simulink model "distmodelR2019a"  (R2019a)
settings: Solver=FixedStepAuto  StartTime=0.0  StopTime=t_sim  FixedStep=TimeStep  RelTol=1e-3
values from neighbouring files (symbols this model uses):
  alt = 300    [main_disturbances_Z.m]
  AX = 0.022    [calctorque.m]    (also in main_disturbances_Z.m)
  AY = 0.034    [calctorque.m]    (also in main_disturbances_Z.m)
  AZ = 0.0748    [calctorque.m]    (also in main_disturbances_Z.m = 0.2108)
  AZES = 0.1156    [calctorque.m]    (also in main_disturbances_Z.m)
  Cdrag = 2.6    [disturbanceCode.m]    (also in main_disturbances_Z.m)
  CLS = [0,-0.195,0.05]    [calctorque.m]    (also in main_disturbances_Z.m)
  Cmy = [0,-0.11,0]    [calctorque.m]    (also in main_disturbances_Z.m)
  CRS = [0,0.195,0.05]    [calctorque.m]    (also in main_disturbances_Z.m)
  D = [-0.17,0.11,0.05]    [projectionTorque1.m]    (also in projectionTorque1_comment.m; projectionTorque2.m; projectionTorque3.m = [-0.17,-0.11,0.05]; projectionTorque4.m = [-0.17,-0.11,0.05])
  ESS = 0.0578    [calctorque.m]    (also in main_disturbances_Z.m)
  G = [OGX,OGY,OGZ]    [disturbanceCode.m]    (also in main_disturbances_Z.m)
  inc = rad2deg(inc)    [main_disturbances_Z.m]
  nmax = 2    [main_disturbances_Z.m]
  nu = rad2deg(nu)    [main_disturbances_Z.m]
  OGX = 2.5*1e-3    (= 0.0025)    [disturbanceCode.m]    (also in main_disturbances_Z.m)
  OGY = 1*1e-2    (= 0.01)    [disturbanceCode.m]    (also in main_disturbances_Z.m = -0.01)
  OGZ = 1*1e-2    (= 0.01)    [disturbanceCode.m]    (also in main_disturbances_Z.m = -0.02)
  OX = 0.17    [calctorque.m]    (also in main_disturbances_Z.m)
  OY = 0.11    [calctorque.m]    (also in main_disturbances_Z.m)
  OZ = 0.05    [calctorque.m]    (also in main_disturbances_Z.m)
  RAAN = rad2deg(RAAN)    [main_disturbances_Z.m]
  RSD = [0.08,0.08,0.08]    [main_disturbances_Z.m]
  Use_IGRF = 0    [main_disturbances_Z.m]
  w = rad2deg(w)    [main_disturbances_Z.m]
undefined symbols (not defined in the file or in its folder): date, DipoleMod, ecc, km, s
libraries: vrlib x19, dspmathops x6, sharedtransform x4, aerolibutil x4, dspindex x3, aerolibconvert2 x2, simulink_extras x1, aerolibatmos2 x1, aerolibcelestial x1, sharedutil x1, aerolibgravity2 x1
(part 2 of 2)

== matlab function distmodelR2019a/Disturbance Torques /drag_torque/here we take care of the shadowing /If Action Subsystem2/MATLAB Function ==
  data: G input; yy output; vorbit input
function yy = fcn(G, vorbit)
% les 4 points qui delimite le cadre 2
A=[0.17,0.11,0.05];%ok
B=[0.17,0.11,-0.05];
C=[-0.17,0.11,-0.05];
D=[-0.17,0.11,0.05];%ok


torque=[0,0,0];
%projection of B
pBz=0.05;
t=(pBz-B(3))/vorbit(3);
pBx=B(1)+t*vorbit(1);
pBy=B(2)+t*vorbit(2);

%projection of c
pCz=pBz;
pCx=C(1)+t*vorbit(1);%% 
pCy=pBy;%% because the projection is in this case //
%vecteur directeur de notre droite
ux=A(1)-pBx;
uy=A(2)-pBy;
uz=A(3)-pBz;

if pCy<0.28
    if pBx<0.17
        
        if pBx>-0.17 %%we caculate(frcement pCx<-0.17)
            %pas
            N=100;%%%%%%%%%%%%%%%%%%%can be changed
            pas=ux/N;
            %integrale de rieman
      
            for i=0:N-1
                xr=pBx+i*pas;
                t=(xr-A(1))/ux;
                y=A(2)+t*uy;
                %geometric center for dA
                Gc=[xr+(pas/2),(0.28+y)/2,pBz];
                Rs=Gc-G;
                torque= torque +cross(Rs,vorbit)*((0.28-y)*pas);
            end
            %the other surface
            Gc=[(pBx-0.17)/2,(pBy+0.28)/2,pBz];
            Rs=Gc-G;
            torque=torque+(pBx+0.17)*(0.28-pBy)*cross(Rs,vorbit);
        else
            %%we calculate(la droite (ApB) coupe [segment]
            N=200;
            pas=0.34/N;
            
            for i=0:N-1
                xr=-0.17+i*pas;
                t=(xr-A(1))/ux;
                y=A(2)+t*uy;
                Gc=[xr+(pas/2),(y+0.28)/2,pBz];
                Rs=Gc-G;
                torque= torque +cross(Rs,vorbit)*((0.28-y)*pas);
                
            end
            
            
            
        end
        
    elseif pCx<0.17 %%we konw already that pCx>-0.17
        %we calculate
        ux=D(1)-pCx;
        uy=D(2)-pCy;
        uz=D(3)-pCz;
        N=100;
        pas=ux/N;%negative always
       
        for i=0:N-1
            xr=pCx+i*pas;
            t=(xr-D(1))/ux;
            y=D(2)+t*uy;
            %geometric center for dA
            Gc=[xr+(pas/2),(y+0.28)/2,pCz];
            Rs=Gc-G;
            torque= torque +cross(Rs,vorbit)*((0.28-y)*pas);
            
        end
        Gc=[(pCx+0.17)/2,(pCy+0.28)/2,pCz];
        Rs=Gc-G;
        torque=torque+(0.17-pCx)*(0.28-pCy)*cross(Rs,vorbit);
    else
        ux=D(1)-pCx;
        uy=D(2)-pCy;
        uz=D(3)-pCz;
        %we calculate(coupe droite segment)
        N=200;
        pas=-0.34/N;
     
        for i=0:N-1
            xr=0.17+i*pas;
            t=(xr-D(1))/ux;
            y=D(2)+t*uy;
            Gc=[xr+(pas/2),(y+0.28)/2,pCz];
            Rs=Gc-G;
            torque= torque +cross(Rs,vorbit)*((0.28-y)*pas);
            
        end
        
    end
else
    %let Dprim Aprim to be like
    Dprim=[-0.17,0.28,0.05];
    Aprim=[0.17,0.28,0.05];
    if pBx<0.17
        ux=A(1)-pBx;
        uy=A(2)-pBy;
        uz=A(3)-pBz;
        %%%%
        ADpv=A-Dprim;
        %%%%%
        tprim=(pBy-A(2))/ADpv(2);
        %on compare
        xc=A(1)+tprim*ADpv(1);
        if pBx<xc%%%derriere suivant les x negative
            N=200;%%%%%%%%%%%%%%%%%%%can be changed
            pas=0.34/N;
            %integrale de rieman
            
            for i=0:N-1
                xr=-0.17+i*pas;%%%intersection DDprim
                t=(xr-A(1))/ux;
                y=A(2)+t*uy;
                %geometric center for dA
                Gc=[xr+(pas/2),(y+0.28)/2,pBz];
                Rs=Gc-G;
                torque= torque +cross(Rs,vorbit)*((0.28-y)*pas);
            end
            
        else
            %we calculate%%%%%%%%%%problem(we can use diagonale)
            t=(0.28-A(2))/uy;%%intersection DprimAprim
            x=A(1)+t*ux;
            N=100;%%%%%%%%%%%%%%%%%%%can be changed
            pas=(0.17-x)/N;
            %integrale de rieman
          
            for i=0:N-1
                xr=x+i*pas;
                t=(xr-A(1))/ux;
                y=A(2)+t*uy;
                %geometric center for dA
                Gc=[xr+(pas/2),(y+0.28)/2,pBz];
                Rs=Gc-G;
                torque= torque +cross(Rs,vorbit)*((0.28-y)*pas);
            end
            
            
            
        end
        %%elseif pCx<0.17
        %we calculate
    else
        ux=D(1)-pCx;
        uy=D(2)-pCy;
        uz=D(3)-pCz;
        %%%%
        DApv=D-Aprim;
        %%%%%
        tprim=(pCy-A(2))/DApv(2);
        %on compare
        xc=D(1)+tprim*DApv(1);
        
        if pCx>xc
            N=200;%%%%%%%%%%%%%%%%%%%can be changed
            pas=-0.34/N;
            %integrale de rieman
            
            for i=0:N-1
                xr=0.17+i*pas;
                t=(xr-D(1))/ux;
                y=D(2)+t*uy;
                %geometric center for dA
                Gc=[xr+(pas/2),(y+0.28)/2,pCz];
                Rs=Gc-G;
                torque= torque +cross(Rs,vorbit)*((0.28-y)*pas);
            end
            
        else
            %we calculate%%%%%%%%%%problem(we can use diagonale)
            t=(0.28-D(2))/uy;
            x=D(1)+t*ux;
            N=100;%%%%%%%%%%%%%%%%%%%can be changed
            pas=(-0.17-x)/N;
            %integrale de rieman
           
            for i=0:N-1
                xr=x+i*pas;
                t=(xr-D(1))/ux;
                y=D(2)+t*uy;
                %geometric center for dA
                Gc=[xr+(pas/2),(y+0.28)/2,pCz];
                Rs=Gc-G;
                torque= torque +cross(Rs,vorbit)*((0.28-y)*pas);
            end
            
            
            
        end
        
    end
    
end
yy=torque;

== matlab function distmodelR2019a/Disturbance Torques /drag_torque/here we take care of the shadowing /If Action Subsystem3/MATLAB Function ==
  data: G input; vorbit input; y output
function y = fcn(G, vorbit)
% les 4 points qui delimite le cadre 1
A=[0.17,-0.11,0.05];%ok
B=[0.17,-0.28,0.05];
C=[-0.17,-0.28,0.05];
D=[-0.17,-0.11,0.05];%ok


torque=[0,0,0];


%projection of B
pBy=-0.11;
t=(pBy-B(2))/vorbit(2);
pBx=B(1)+t*vorbit(1);
pBz=B(3)+t*vorbit(3);

%projection of c
pCy=pBy;
pCx=C(1)+t*vorbit(1);%% because they have the same y
pCz=pBz;
%vecteur directeur de notre droite
ux=A(1)-pBx;
uy=A(2)-pBy;
uz=A(3)-pBz;
if pCz>-0.05
    if pBx<0.17
        
        if pBx>-0.17 %%we caculate(frcement pCx<-0.17)
            %pas
            N=100;%%%%%%%%%%%%%%%%%%%can be changed
            pas=ux/N;
            %integrale de rieman
            for i=0:N-1
                xr=pBx+i*pas;
                t=(xr-A(1))/ux;
                z=A(3)+t*uz;
                %geometric center for dA
                Gc=[xr+(pas/2),pBy,(z-0.05)/2];
                Rs=Gc-G;
                torque= torque +cross(Rs,vorbit)*((z+0.05)*pas);
            end
            %the other surface
            Gc=[(pBx-0.17)/2,pBy,(pBz-0.05)/2];
            Rs=Gc-G;
            torque=torque+(pBx+0.17)*(pBz+0.05)*cross(Rs,vorbit);
        else
            %%we calculate(la droite (ApB) coupe [segment]
            N=200;
            pas=0.34/N;
            
            for i=0:N-1
                xr=-0.17+i*pas;
                t=(xr-A(1))/ux;
                z=A(3)+t*uz;
                Gc=[xr+(pas/2),pBy,(z-0.05)/2];
                Rs=Gc-G;
                torque= torque +cross(Rs,vorbit)*((z+0.05)*pas);
                
            end
            
            
            
        end
        
    elseif pCx<0.17 %%we konw already that pCx>-0.17
        %we calculate
        ux=D(1)-pCx;
        uy=D(2)-pCy;
        uz=D(3)-pCz;
        N=100;
        pas=ux/N;%negative always
       
        for i=0:N-1
            xr=pCx+i*pas;
            t=(xr-D(1))/ux;
            z=D(3)+t*uz;
            %geometric center for dA
            Gc=[xr+(pas/2),pCy,(z-0.05)/2];
            Rs=Gc-G;
            torque= torque +cross(Rs,vorbit)*((z+0.05)*pas);
            
        end
        Gc=[(pCx+0.17)/2,pCy,(pCz-0.05)/2];
        Rs=Gc-G;
        torque=torque+(0.17-pCx)*(pCz+0.05)*cross(Rs,vorbit);
    else
        ux=D(1)-pCx;
        uy=D(2)-pCy;
        uz=D(3)-pCz;
        %we calculate(coupe droite segment)
        N=200;
        pas=-0.34/N;
     
        for i=0:N-1
            xr=0.17+i*pas;
            t=(xr-D(1))/ux;
            z=D(3)+t*uz;
            Gc=[xr+(pas/2),pCy,(z-0.05)/2];
            Rs=Gc-G;
            torque= torque +cross(Rs,vorbit)*((z+0.05)*pas);
            
        end
        
    end
else
    %let Dprim Aprim to be like
    Dprim=[-0.17,-0.11,-0.05];
    Aprim=[0.17,-0.11,-0.05];
    if pBx<0.17
        ux=A(1)-pBx;
        uy=A(2)-pBy;
        uz=A(3)-pBz;
        %%%%
        ADpv=A-Dprim;
        %%%%%
        tprim=(pBz-A(3))/ADpv(3);
        %on compare
        xc=A(1)+tprim*ADpv(1);
        if pBx<xc%%%derriere suivant les x negative
            N=200;%%%%%%%%%%%%%%%%%%%can be changed
            pas=0.34/N;
            %integrale de rieman
            
            for i=0:N-1
                xr=-0.17+i*pas;%%%intersection DDprim
                t=(xr-A(1))/ux;
                z=A(3)+t*uz;
                %geomretric center for dA
                Gc=[xr+(pas/2),pBy,(z-0.05)/2];
                Rs=Gc-G;
                torque= torque +cross(Rs,vorbit)*((z+0.05)*pas);
            end
            
        else
            %we calculate%%%%%%%%%%problem(we can use diagonale)
            t=(-0.05-A(3))/uz;%%intersection DprimAprim
            x=A(1)+t*ux;
            N=100;%%%%%%%%%%%%%%%%%%%can be changed
            pas=(0.17-x)/N;
            %integrale de rieman
          
            for i=0:N-1
                xr=x+i*pas;
                t=(xr-A(1))/ux;
                z=A(3)+t*uz;
                %geometric center for dA
                Gc=[xr+(pas/2),pBy,(z-0.05)/2];
                Rs=Gc-G;
                torque= torque +cross(Rs,vorbit)*((z+0.05)*pas);
            end
            
            
            
        end
        %%elseif pCx<0.17
        %we calculate
    else
        ux=D(1)-pCx;
        uy=D(2)-pCy;
        uz=D(3)-pCz;
        %%%%
        DApv=D-Aprim;
        %%%%%
        tprim=(pCz-A(3))/DApv(3);
        %on compare
        xc=D(1)+tprim*DApv(1);
        
        if pCx>xc
            N=200;%%%%%%%%%%%%%%%%%%%can be changed
            pas=-0.34/N;
            %integrale de rieman
            
            for i=0:N-1
                xr=0.17+i*pas;
                t=(xr-D(1))/ux;
                z=D(3)+t*uz;
                %geometric center for dA
                Gc=[xr+(pas/2),pCy,(z-0.05)/2];
                Rs=Gc-G;
                torque= torque +cross(Rs,vorbit)*((z+0.05)*pas);
            end
            
        else
            %we calculate%%%%%%%%%%problem(we can use diagonale)
            t=(-0.05-D(3))/uz;
            x=D(1)+t*ux;
            N=100;%%%%%%%%%%%%%%%%%%%can be changed
            pas=(-0.17-x)/N;
            %integrale de rieman
           
            for i=0:N-1
                xr=x+i*pas;
                t=(xr-D(1))/ux;
                z=D(3)+t*uz;
                %geometric center for dA
                Gc=[xr+(pas/2),pBy,(z-0.05)/2];
                Rs=Gc-G;
                torque= torque +cross(Rs,vorbit)*((z+0.05)*pas);
            end
            
            
            
        end
        
    end
    
end
y=torque;

== matlab function distmodelR2019a/Disturbance Torques /drag_torque/here we take care of the shadowing /If Action Subsystem4/MATLAB Function ==
  data: G input; yy output; vorbit input
function yy = fcn(G, vorbit)
% les 4 points qui delimite le cadre 2
A=[0.17,-0.11,0.05];%ok
B=[0.17,-0.11,-0.05];
C=[-0.17,-0.11,-0.05];
D=[-0.17,-0.11,0.05];%ok


torque=[0,0,0];
%projection of B
pBz=0.05;
t=(pBz-B(3))/vorbit(3);
pBx=B(1)+t*vorbit(1);
pBy=B(2)+t*vorbit(2);

%projection of c
pCz=pBz;
pCx=C(1)+t*vorbit(1);%% 
pCy=pBy;%% because the projection is in this case //
%vecteur directeur de notre droite
ux=A(1)-pBx;
uy=A(2)-pBy;
uz=A(3)-pBz;

if pCy>-0.28
    if pBx<0.17
        
        if pBx>-0.17 %%we caculate(frcement pCx<-0.17)
            %pas
            N=100;%%%%%%%%%%%%%%%%%%%can be changed
            pas=ux/N;
            %integrale de rieman
      
            for i=0:N-1
                xr=pBx+i*pas;
                t=(xr-A(1))/ux;
                y=A(2)+t*uy;
                %geometric center for dA
                Gc=[xr+(pas/2),(-0.28+y)/2,pBz];
                Rs=Gc-G;
                torque= torque +cross(Rs,vorbit)*((y+0.28)*pas);
            end
            %the other surface
            Gc=[(pBx-0.17)/2,(pBy-0.28)/2,pBz];
            Rs=Gc-G;
            torque=torque+(pBx+0.17)*(pBy+0.28)*cross(Rs,vorbit);
        else
            %%we calculate(la droite (ApB) coupe [segment]
            N=200;
            pas=0.34/N;
            
            for i=0:N-1
                xr=-0.17+i*pas;
                t=(xr-A(1))/ux;
                y=A(2)+t*uy;
                Gc=[xr+(pas/2),(y-0.28)/2,pBz];
                Rs=Gc-G;
                torque= torque +cross(Rs,vorbit)*((y+0.28)*pas);
                
            end
            
            
            
        end
        
    elseif pCx<0.17 %%we konw already that pCx>-0.17
        %we calculate
        ux=D(1)-pCx;
        uy=D(2)-pCy;
        uz=D(3)-pCz;
        N=100;
        pas=ux/N;%negative always
       
        for i=0:N-1
            xr=pCx+i*pas;
            t=(xr-D(1))/ux;
            y=D(2)+t*uy;
            %geometric center for dA
            Gc=[xr+(pas/2),(y-0.28)/2,pCz];
            Rs=Gc-G;
            torque= torque +cross(Rs,vorbit)*((y+0.28)*pas);
            
        end
        Gc=[(pCx+0.17)/2,(pCy-0.28)/2,pCz];
        Rs=Gc-G;
        torque=torque+(0.17-pCx)*(pCy+0.28)*cross(Rs,vorbit);
    else
        ux=D(1)-pCx;
        uy=D(2)-pCy;
        uz=D(3)-pCz;
        %we calculate(coupe droite segment)
        N=200;
        pas=-0.34/N;
     
        for i=0:N-1
            xr=0.17+i*pas;
            t=(xr-D(1))/ux;
            y=D(2)+t*uy;
            Gc=[xr+(pas/2),(y-0.28)/2,pCz];
            Rs=Gc-G;
            torque= torque +cross(Rs,vorbit)*((y+0.28)*pas);
            
        end
        
    end
else
    %let Dprim Aprim to be like
    Dprim=[-0.17,-0.28,0.05];
    Aprim=[0.17,-0.28,0.05];
    if pBx<0.17
        ux=A(1)-pBx;
        uy=A(2)-pBy;
        uz=A(3)-pBz;
        %%%%
        ADpv=A-Dprim;
        %%%%%
        tprim=(pBy-A(2))/ADpv(2);
        %on compare
        xc=A(1)+tprim*ADpv(1);
        if pBx<xc%%%derriere suivant les x negative
            N=200;%%%%%%%%%%%%%%%%%%%can be changed
            pas=0.34/N;
            %integrale de rieman
            
            for i=0:N-1
                xr=-0.17+i*pas;%%%intersection DDprim
                t=(xr-A(1))/ux;
                y=A(2)+t*uy;
                %geometric center for dA
                Gc=[xr+(pas/2),(y-0.28)/2,pBz];
                Rs=Gc-G;
                torque= torque +cross(Rs,vorbit)*((y+0.28)*pas);
            end
            
        else
            %we calculate%%%%%%%%%%problem(we can use diagonale)
            t=(-0.28-A(2))/uy;%%intersection DprimAprim
            x=A(1)+t*ux;
            N=100;%%%%%%%%%%%%%%%%%%%can be changed
            pas=(0.17-x)/N;
            %integrale de rieman
          
            for i=0:N-1
                xr=x+i*pas;
                t=(xr-A(1))/ux;
                y=A(2)+t*uy;
                %geometric center for dA
                Gc=[xr+(pas/2),(y-0.28)/2,pBz];
                Rs=Gc-G;
                torque= torque +cross(Rs,vorbit)*((y+0.28)*pas);
            end
            
            
            
        end
        %%elseif pCx<0.17
        %we calculate
    else
        ux=D(1)-pCx;
        uy=D(2)-pCy;
        uz=D(3)-pCz;
        %%%%
        DApv=D-Aprim;
        %%%%%
        tprim=(pCy-A(2))/DApv(2);
        %on compare
        xc=D(1)+tprim*DApv(1);
        
        if pCx>xc
            N=200;%%%%%%%%%%%%%%%%%%%can be changed
            pas=-0.34/N;
            %integrale de rieman
            
            for i=0:N-1
                xr=0.17+i*pas;
                t=(xr-D(1))/ux;
                y=D(2)+t*uy;
                %geometric center for dA
                Gc=[xr+(pas/2),(y-0.28)/2,pCz];
                Rs=Gc-G;
                torque= torque +cross(Rs,vorbit)*((y+0.28)*pas);
            end
            
        else
            %we calculate%%%%%%%%%%problem(we can use diagonale)
            t=(-0.28-D(2))/uy;
            x=D(1)+t*ux;
            N=100;%%%%%%%%%%%%%%%%%%%can be changed
            pas=(-0.17-x)/N;
            %integrale de rieman
           
            for i=0:N-1
                xr=x+i*pas;
                t=(xr-D(1))/ux;
                y=D(2)+t*uy;
                %geometric center for dA
                Gc=[xr+(pas/2),(y-0.28)/2,pCz];
                Rs=Gc-G;
                torque= torque +cross(Rs,vorbit)*((y+0.28)*pas);
            end
            
            
            
        end
        
    end
    
end
yy=torque;

== matlab function distmodelR2019a/Time propagator/MATLAB Function ==
  data: t input; Y output; DOY output; S output
function [Y, DOY, S] = DOY(t)
Y = 2022 + fix(t/31557600);
DOY = 1+fix((t-floor(t/31557600)*31557600)/86400);
S = t - fix(t/31557600)*31557600 - (DOY-1)*86400;
